simulink model "new_ass13"  (R2023a)
settings: Solver=VariableStepAuto  StartTime=0.0  StopTime=10.0  RelTol=1e-3
undefined symbols (not defined in the file): dqi, K, KD, KDt, KP, KPt, Mt, qi, robot, xr
settings Model: Creator=franc  LastModifiedBy=franc

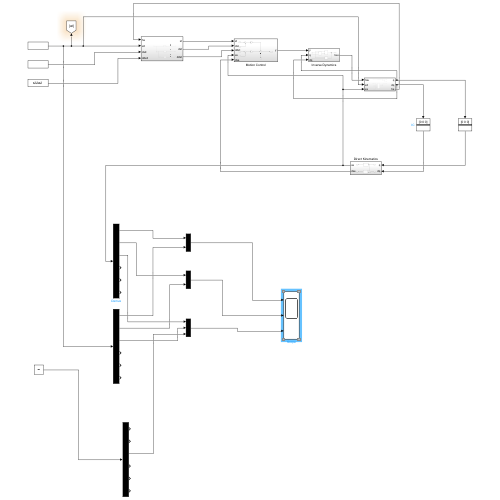
[thumbnail: Simulink's stored preview of the top-level diagram]
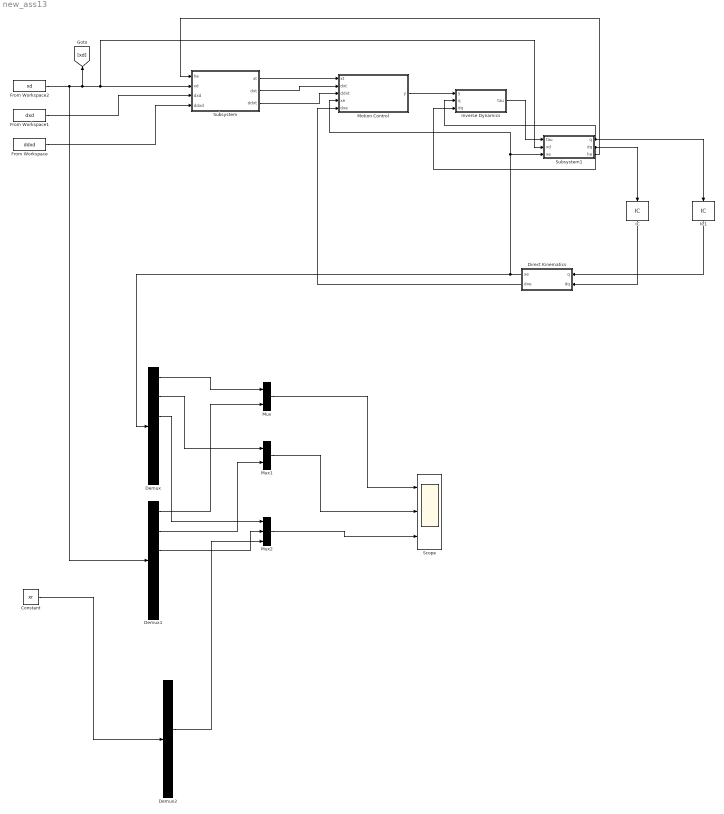
== system new_ass13 ==
  Constant : Constant  Value=xr
  Demux : Demux  Outputs=6
  Demux1 : Demux  Outputs=6
  Demux2 : Demux  Outputs=6
  Direct Kinematics : Subsystem
  From Workspace : FromWorkspace  VariableName=ddxd
  From Workspace1 : FromWorkspace  VariableName=dxd
  From Workspace2 : FromWorkspace  VariableName=xd
  IC : InitialCondition  Value=[0 0 0]
  IC1 : InitialCondition  Value=[0 0 0]
  Inverse Dynamics : Subsystem
  Motion Control : Subsystem
  Mux : Mux  Inputs=2
  Mux1 : Mux  Inputs=2
  Mux2 : Mux  Inputs=3
  Scope : Scope  NumInputPorts=3
  Subsystem : Subsystem
  Subsystem1 : Subsystem
  wires:
  From Workspace/1 -> Subsystem/4(ddxd)
  From Workspace1/1 -> Subsystem/3(dxd)
  From Workspace2/1 -> Demux1/1, Subsystem1/2(xd), Subsystem/2(xd), [xd]
  Subsystem/1(xt) -> Motion Control/1(xt)
  Subsystem/2(dxt) -> Motion Control/2(dxt)
  Subsystem/3(ddxt) -> Motion Control/3(ddxt)
  Motion Control/1(y) -> Inverse Dynamics/1(y)
  Inverse Dynamics/1(tau) -> Subsystem1/1(tau)
  Subsystem1/1(q) -> Inverse Dynamics/2(q), IC1/1
  Subsystem1/2(dq) -> Inverse Dynamics/3(dq), IC/1
  Direct Kinematics/1(xe) -> Demux/1, Motion Control/4(xe), Subsystem1/3(xe)
  Direct Kinematics/2(dxe) -> Motion Control/5(dxe)
  Subsystem1/3(he) -> Subsystem/1(he)
  IC/1 -> Direct Kinematics/2(dq)
  IC1/1 -> Direct Kinematics/1(q)
  Demux/1 -> Mux/1
  Demux1/1 -> Mux/2
  Demux/2 -> Mux1/1
  Demux1/2 -> Mux1/2
  Demux/3 -> Mux2/1
  Demux1/3 -> Mux2/2
  Mux/1 -> Scope/1
  Mux1/1 -> Scope/2
  Mux2/1 -> Scope/3
  Constant/1 -> Demux2/1
  Demux2/3 -> Mux2/3

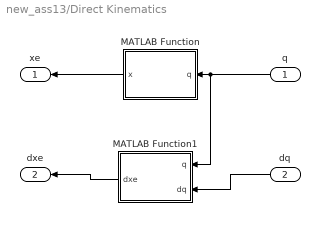
== system new_ass13/Direct Kinematics ==
  q : Inport
  dq : Inport  Port=2
  MATLAB Function : MATLAB Function  TreatAsAtomicUnit=on
  MATLAB Function1 : MATLAB Function  TreatAsAtomicUnit=on
  xe : Outport
  dxe : Outport  Port=2
  wires:
  q/1 -> MATLAB Function1/1(q), MATLAB Function/1(q)
  MATLAB Function/1(x) -> xe/1
  MATLAB Function1/1(dxe) -> dxe/1
  dq/1 -> MATLAB Function1/2(dq)

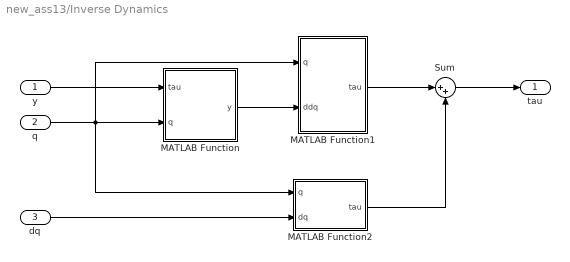
== system new_ass13/Inverse Dynamics ==
  y : Inport
  q : Inport  Port=2
  dq : Inport  Port=3
  MATLAB Function : MATLAB Function  TreatAsAtomicUnit=on
  MATLAB Function1 : MATLAB Function  TreatAsAtomicUnit=on
  MATLAB Function2 : MATLAB Function  TreatAsAtomicUnit=on
  Sum : Sum  Inputs=|++
  tau : Outport
  wires:
  Sum/1 -> tau/1
  MATLAB Function2/1(tau) -> Sum/2
  MATLAB Function1/1(tau) -> Sum/1
  dq/1 -> MATLAB Function2/2(dq)
  MATLAB Function/1(y) -> MATLAB Function1/2(ddq)
  q/1 -> MATLAB Function1/1(q), MATLAB Function2/1(q), MATLAB Function/2(q)
  y/1 -> MATLAB Function/1(tau)

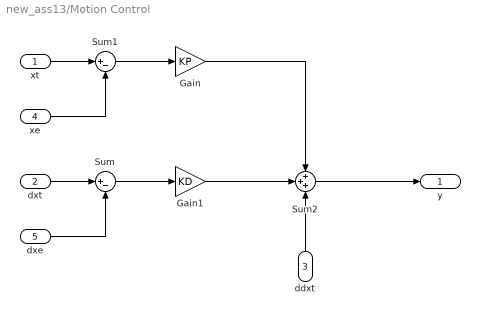
== system new_ass13/Motion Control ==
  xt : Inport
  dxt : Inport  Port=2
  ddxt : Inport  Port=3
  xe : Inport  Port=4
  dxe : Inport  Port=5
  Gain : Gain  Gain=KP
  Gain1 : Gain  Gain=KD
  Sum : Sum  Inputs=|+-
  Sum1 : Sum  Inputs=|+-
  Sum2 : Sum  Inputs=+++
  y : Outport
  wires:
  ddxt/1 -> Sum2/3
  Gain1/1 -> Sum2/2
  Gain/1 -> Sum2/1
  Sum2/1 -> y/1
  Sum1/1 -> Gain/1
  Sum/1 -> Gain1/1
  xt/1 -> Sum1/1
  xe/1 -> Sum1/2
  dxe/1 -> Sum/2
  dxt/1 -> Sum/1

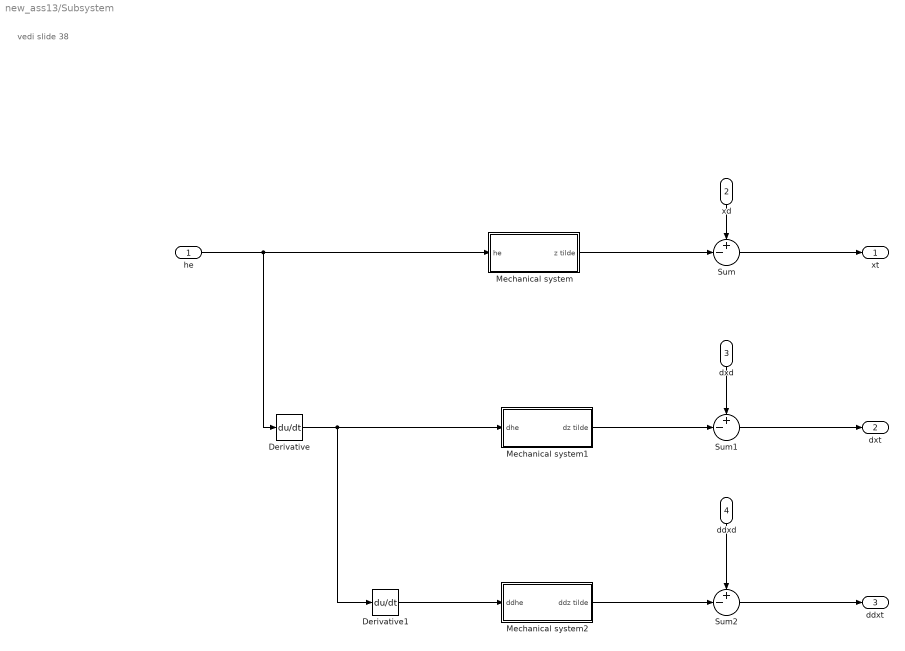
== system new_ass13/Subsystem ==
  note: vedi slide 38
  he : Inport
  xd : Inport  Port=2
  dxd : Inport  Port=3
  ddxd : Inport  Port=4
  Derivative : Derivative
  Derivative1 : Derivative
  Mechanical system : Subsystem
  Mechanical system1 : Subsystem
  Mechanical system2 : Subsystem
  Sum : Sum  Inputs=+-|
  Sum1 : Sum  Inputs=+-|
  Sum2 : Sum  Inputs=+-|
  xt : Outport
  dxt : Outport  Port=2
  ddxt : Outport  Port=3
  wires:
  Sum/1 -> xt/1
  Mechanical system2/1(ddz tilde) -> Sum2/2
  Derivative1/1 -> Mechanical system2/1(ddhe)
  Mechanical system1/1(dz tilde) -> Sum1/2
  Mechanical system/1(z tilde) -> Sum/2
  Derivative/1 -> Derivative1/1, Mechanical system1/1(dhe)
  Sum2/1 -> ddxt/1
  ddxd/1 -> Sum2/1
  Sum1/1 -> dxt/1
  dxd/1 -> Sum1/1
  he/1 -> Derivative/1, Mechanical system/1(he)
  xd/1 -> Sum/1

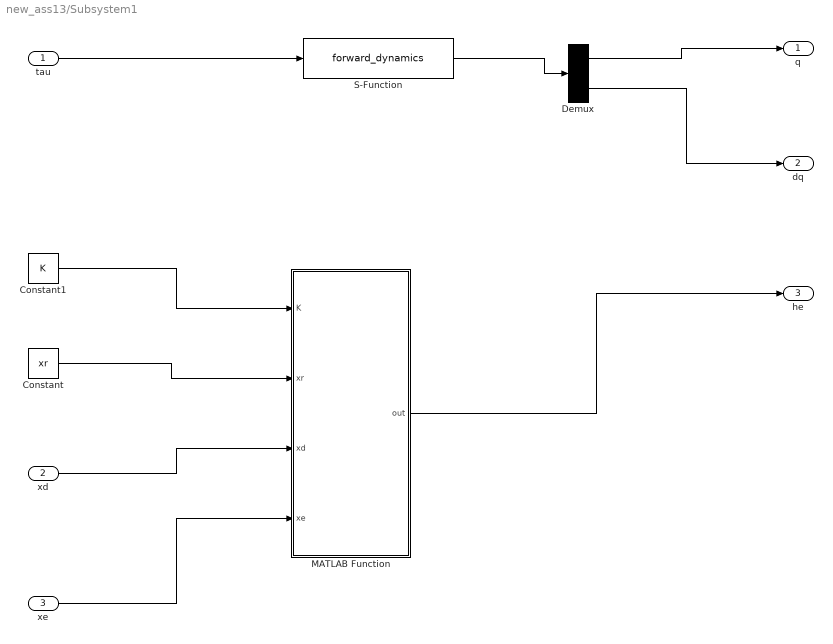
== system new_ass13/Subsystem1 ==
  tau : Inport
  xd : Inport  Port=2
  xe : Inport  Port=3
  Constant : Constant  Value=xr
  Constant1 : Constant  Value=K
  Demux : Demux  Outputs=2
  MATLAB Function : MATLAB Function  TreatAsAtomicUnit=on
  S-Function : S-Function  FunctionName=forward_dynamics  Parameters=robot,qi,dqi  SFunctionDeploymentMode=off  EnableBusSupport=off
  q : Outport
  dq : Outport  Port=2
  he : Outport  Port=3
  wires:
  tau/1 -> S-Function/1
  S-Function/1 -> Demux/1
  Demux/1 -> q/1
  Demux/2 -> dq/1
  Constant1/1 -> MATLAB Function/1(K)
  Constant/1 -> MATLAB Function/2(xr)
  xd/1 -> MATLAB Function/3(xd)
  xe/1 -> MATLAB Function/4(xe)
  MATLAB Function/1(out) -> he/1

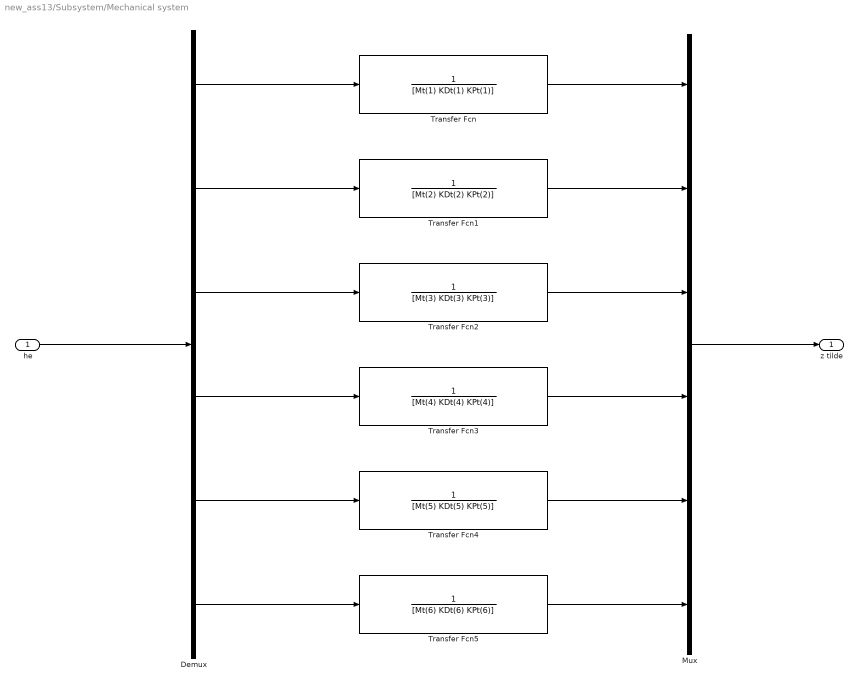
== system new_ass13/Subsystem/Mechanical system ==
  he : Inport
  Demux : Demux  Outputs=6
  Mux : Mux  Inputs=6
  Transfer Fcn : TransferFcn  Denominator=[Mt(1) KDt(1) KPt(1)]
  Transfer Fcn1 : TransferFcn  Denominator=[Mt(2) KDt(2) KPt(2)]
  Transfer Fcn2 : TransferFcn  Denominator=[Mt(3) KDt(3) KPt(3)]
  Transfer Fcn3 : TransferFcn  Denominator=[Mt(4) KDt(4) KPt(4)]
  Transfer Fcn4 : TransferFcn  Denominator=[Mt(5) KDt(5) KPt(5)]
  Transfer Fcn5 : TransferFcn  Denominator=[Mt(6) KDt(6) KPt(6)]
  z tilde : Outport
  wires:
  Mux/1 -> z tilde/1
  Transfer Fcn4/1 -> Mux/5
  Transfer Fcn5/1 -> Mux/6
  Transfer Fcn3/1 -> Mux/4
  Transfer Fcn2/1 -> Mux/3
  Transfer Fcn1/1 -> Mux/2
  Transfer Fcn/1 -> Mux/1
  Demux/6 -> Transfer Fcn5/1
  Demux/5 -> Transfer Fcn4/1
  Demux/4 -> Transfer Fcn3/1
  Demux/2 -> Transfer Fcn1/1
  Demux/3 -> Transfer Fcn2/1
  Demux/1 -> Transfer Fcn/1
  he/1 -> Demux/1

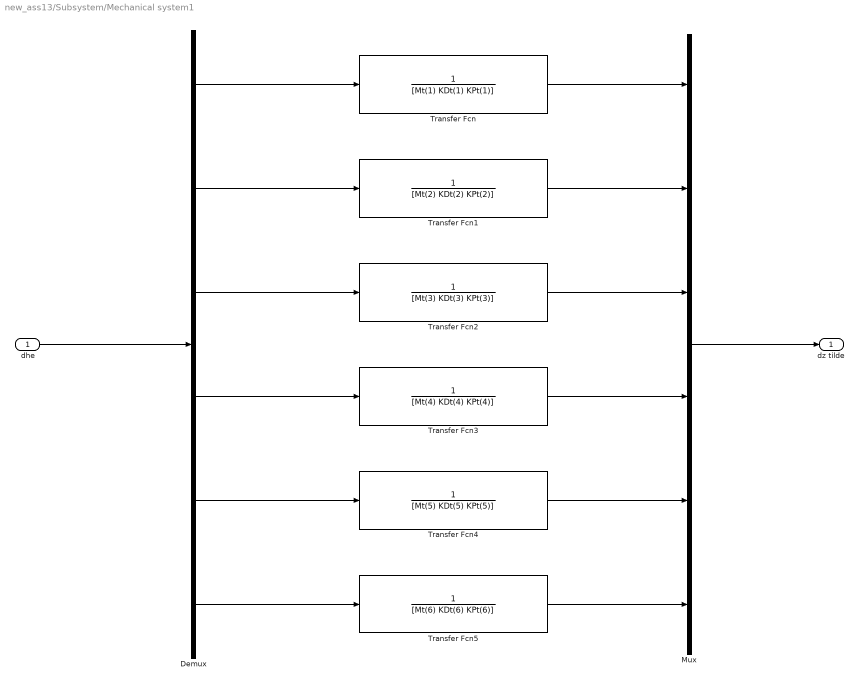
== system new_ass13/Subsystem/Mechanical system1 ==
  dhe : Inport
  Demux : Demux  Outputs=6
  Mux : Mux  Inputs=6
  Transfer Fcn : TransferFcn  Denominator=[Mt(1) KDt(1) KPt(1)]
  Transfer Fcn1 : TransferFcn  Denominator=[Mt(2) KDt(2) KPt(2)]
  Transfer Fcn2 : TransferFcn  Denominator=[Mt(3) KDt(3) KPt(3)]
  Transfer Fcn3 : TransferFcn  Denominator=[Mt(4) KDt(4) KPt(4)]
  Transfer Fcn4 : TransferFcn  Denominator=[Mt(5) KDt(5) KPt(5)]
  Transfer Fcn5 : TransferFcn  Denominator=[Mt(6) KDt(6) KPt(6)]
  dz tilde : Outport
  wires:
  Mux/1 -> dz tilde/1
  Transfer Fcn4/1 -> Mux/5
  Transfer Fcn5/1 -> Mux/6
  Transfer Fcn3/1 -> Mux/4
  Transfer Fcn2/1 -> Mux/3
  Transfer Fcn1/1 -> Mux/2
  Transfer Fcn/1 -> Mux/1
  Demux/6 -> Transfer Fcn5/1
  Demux/5 -> Transfer Fcn4/1
  Demux/4 -> Transfer Fcn3/1
  Demux/2 -> Transfer Fcn1/1
  Demux/3 -> Transfer Fcn2/1
  Demux/1 -> Transfer Fcn/1
  dhe/1 -> Demux/1

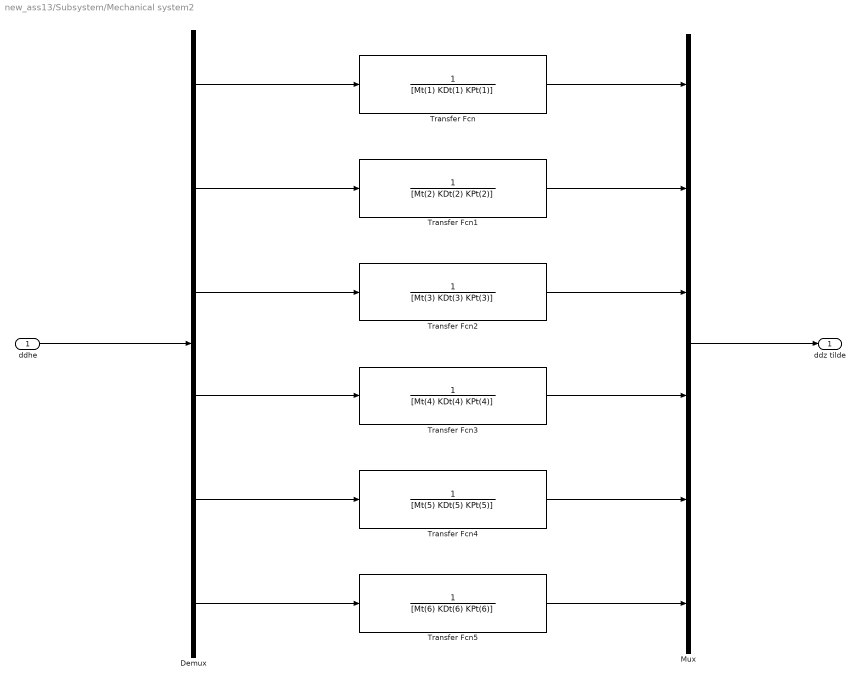
== system new_ass13/Subsystem/Mechanical system2 ==
  ddhe : Inport
  Demux : Demux  Outputs=6
  Mux : Mux  Inputs=6
  Transfer Fcn : TransferFcn  Denominator=[Mt(1) KDt(1) KPt(1)]
  Transfer Fcn1 : TransferFcn  Denominator=[Mt(2) KDt(2) KPt(2)]
  Transfer Fcn2 : TransferFcn  Denominator=[Mt(3) KDt(3) KPt(3)]
  Transfer Fcn3 : TransferFcn  Denominator=[Mt(4) KDt(4) KPt(4)]
  Transfer Fcn4 : TransferFcn  Denominator=[Mt(5) KDt(5) KPt(5)]
  Transfer Fcn5 : TransferFcn  Denominator=[Mt(6) KDt(6) KPt(6)]
  ddz tilde : Outport
  wires:
  Mux/1 -> ddz tilde/1
  Transfer Fcn4/1 -> Mux/5
  Transfer Fcn5/1 -> Mux/6
  Transfer Fcn3/1 -> Mux/4
  Transfer Fcn2/1 -> Mux/3
  Transfer Fcn1/1 -> Mux/2
  Transfer Fcn/1 -> Mux/1
  Demux/6 -> Transfer Fcn5/1
  Demux/5 -> Transfer Fcn4/1
  Demux/4 -> Transfer Fcn3/1
  Demux/2 -> Transfer Fcn1/1
  Demux/3 -> Transfer Fcn2/1
  Demux/1 -> Transfer Fcn/1
  ddhe/1 -> Demux/1

== matlab function new_ass13/Inverse Dynamics/MATLAB Function1 ==
  data: q input; tau output; ddq input
function tau = B(q,ddq)
tau = zeros(3,1);
tau = get_B_as_7(q(1),q(3)) * ddq;

== matlab function new_ass13/Inverse Dynamics/MATLAB Function ==
  data: tau input; y output; q input
function y = JA_inv(tau,q)
y = zeros(3,1);
y = get_Ja_inverse_as_9(q(1),q(2),q(3)) * tau;

== matlab function new_ass13/Inverse Dynamics/MATLAB Function2 ==
  data: q input; tau output; dq input
function tau = n(q,dq)
tau = zeros(3,1);
tau = get_n_as_7(q(1),q(3),dq(1),dq(3));

== matlab function new_ass13/Subsystem1/MATLAB Function ==
  data: K input; out output; xr input; xd input; xe input
function out = environment(K, xr, xd, xe)
%consider the interaction only in z direction
% if the end effector touch the environment 
he = zeros(6,1);

if xe(3) > xr(3)
    %The interaction force between the end-effector and the environment is
    dxrd = xd-xr;
    dxed = xd-xe;
    dxre = dxrd-dxed;
    he = K.*dxre;
end

out = he;

== matlab function new_ass13/Direct Kinematics/MATLAB Function ==
  data: q input; x output
function x = getK(q)

x = new_getK(q);

== matlab function new_ass13/Direct Kinematics/MATLAB Function1 ==
  data: q input; dxe output; dq input
function dxe = Ja(q,dq)

dxe = get_Ja_as_9(q(1),q(2),q(3))*dq;
